simulink model "RC_lowpass"  (R2020a)
settings: Solver=VariableStepAuto  StartTime=0.0  StopTime=10.0  RelTol=1e-3
libraries: simulink x1
settings Model: Creator=Atharv Sharma  LastModifiedBy=Atharv Sharma

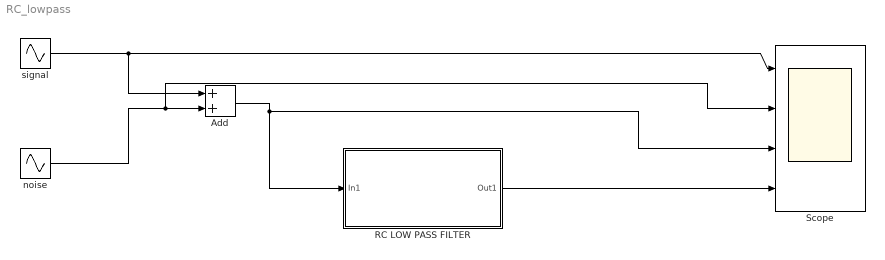
== system RC_lowpass ==
  Add : Sum
  RC LOW PASS FILTER : Subsystem  mask{derivative=1.0}
      mask prompts: derivative "R*C"
      mask TypeOptions derivative: Discrete Derivative/gainval
  Scope : Scope  NumInputPorts=4
  noise : Sin  Amplitude=0.1  Frequency=10  SampleTime=.001
  signal : Sin  Amplitude=5  SampleTime=.001
  wires:
  signal/1 -> Scope/1, Add/1
  noise/1 -> Scope/2, Add/2
  Add/1 -> RC LOW PASS FILTER/1(In1), Scope/3
  RC LOW PASS FILTER/1(Out1) -> Scope/4

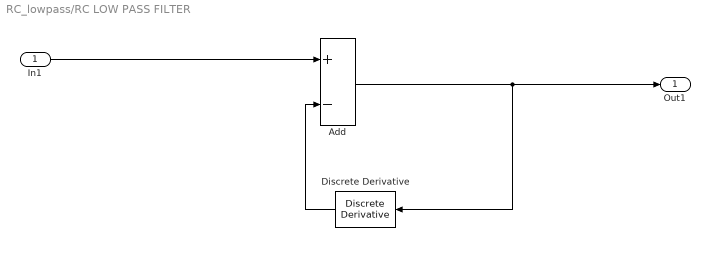
== system RC_lowpass/RC LOW PASS FILTER ==
  In1 : Inport
  Add : Sum  Inputs=+-
  Discrete Derivative : simulink/Discrete/Discrete Derivative  gainval=derivative  ICPrevScaledInput=0.0  OutMin=[]  OutMax=[]  OutDataType=fixdt(1, 16)  OutScaling=2^-10  DoSatur=off
  Out1 : Outport
  wires:
  In1/1 -> Add/1
  Add/1 -> Discrete Derivative/1, Out1/1
  Discrete Derivative/1 -> Add/2
